simulink model "Prob_8_DONE"  (R2025a)
settings: Solver=ode1  StartTime=0.0  StopTime=12  FixedStep=1/360  RelTol=1e-3
settings Model: Creator=claudelieber  LastModifiedBy=yugpn
settings SolverCC: AlgebraicLoopSolver=TrustRegion
settings DataIOCC: ReturnWorkspaceOutputs=off
settings OptimizationCC: ReuseModelBlockBuffer=off
settings DebuggingCC: UnconnectedInputMsg=warning  UnconnectedOutputMsg=warning  UnconnectedLineMsg=warning  ArithmeticOperatorsInVariantConditions=warning
settings ModelReferenceCC: EnableRefExpFcnMdlSchedulingChecks=on
settings SFSimCC: CustomCodeUndefinedFunction=UseInterfaceOnly
settings RTWCC: GPUComputeCapability=3.5  DLArmComputeVersion=19.05

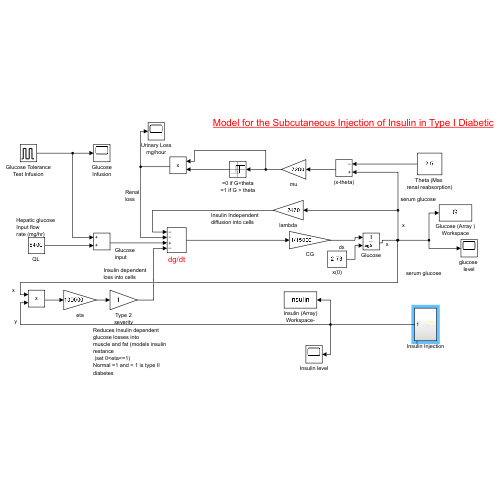
[thumbnail: Simulink's stored preview of the top-level diagram]
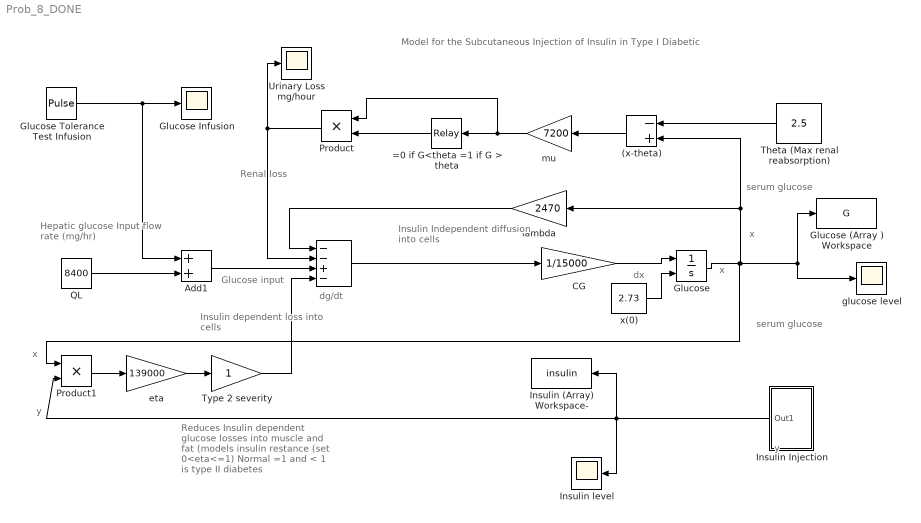
== system Prob_8_DONE ==
  note: Model for the Subcutaneous Injection of Insulin in Type I Diabetic
  note: x
  note: y
  note: y
  note: serum glucose
  note: Reduces Insulin dependent
      | glucose losses into
      | muscle and fat (models insulin
      | restance
      |  (set 0<eta<=1)
      | Normal =1 and < 1 is type II
      | diabetes
  note: x
  note: dx
  note: Insulin dependent
      | loss into cells
  note: serum glucose
  note: dg/dt
  note: Glucose
      | input
  note: x
  note: Renal
      | loss
  note: Insulin Independent
      | diffusion into cells
  note: Hepatic glucose
      | Input flow
      | rate (mg/hr)
  " " : Sum  Inputs=--+-
  (x-theta) : Sum  Inputs=-+
  =0 if G<theta =1 if G > theta : Relay  OnSwitchValue=0  OffSwitchValue=-0.00001
  Add1 : Sum
  CG : Gain  Gain=1/15000
  Glucose : Integrator  InitialConditionSource=external  InitialCondition=0.81
  Glucose Infusion : Scope
      settings: ActiveDisplayYMinimum=-1  ActiveDisplayYMaximum=1  DataLoggingSaveFormat=Array
  Glucose (Array ) Workspace : ToWorkspace  VariableName=G  SampleTime=-1
  Glucose Tolerance Test Infusion : DiscretePulseGenerator  PulseType=Time based  Amplitude=0  Period=10  PulseWidth=5  PhaseDelay=1
  Insulin (Array) Workspace- : ToWorkspace  VariableName=insulin  SampleTime=-1
  Insulin Injection : Subsystem
  Insulin level : Scope
      settings: ActiveDisplayYMinimum=-4.5264238355847652  ActiveDisplayYMaximum=0.89231310643375261  DataLoggingVariableName=ScopeData2  DataLoggingSaveFormat=Array
  Product : Product
  Product1 : Product
  "QL " : Constant  Value=8400
  Theta (Max renal reabsorption) : Constant  Value=2.5
  Type 2 severity : Gain
  Urinary Loss mg/hour : Scope
      settings: ActiveDisplayYMinimum=-1140.6549745940436  ActiveDisplayYMaximum=6361.1676644120716  DataLoggingVariableName=ScopeData3
  "eta " : Gain  Gain=139000
  glucose level : Scope
      settings: ActiveDisplayYMinimum=-26.029411804853417  ActiveDisplayYMaximum=30.5837061812655  DataLoggingSaveFormat=Array
  lambda : Gain  Gain=2470
  mu : Gain  Gain=7200
  x(0) : Constant  Value=2.73
  wires:
  mu/1 -> Product/1, =0 if G<theta =1 if G > theta/1
  " "/1 -> CG/1
  lambda/1 -> " "/1
  Product/1 -> " "/2, Urinary Loss mg/hour/1
  Theta (Max renal reabsorption)/1 -> (x-theta)/1
  x(0)/1 -> Glucose/2
  Glucose/1 -> Product1/1, Glucose (Array ) Workspace/1, glucose level/1, (x-theta)/2, lambda/1
  Product1/1 -> "eta "/1
  Add1/1 -> " "/3
  (x-theta)/1 -> mu/1
  "eta "/1 -> Type 2 severity/1
  =0 if G<theta =1 if G > theta/1 -> Product/2
  Type 2 severity/1 -> " "/4
  CG/1 -> Glucose/1
  "QL "/1 -> Add1/2
  Glucose Tolerance Test Infusion/1 -> Add1/1, Glucose Infusion/1
  Insulin Injection/1(Out1) -> Product1/2, Insulin (Array) Workspace-/1, Insulin level/1

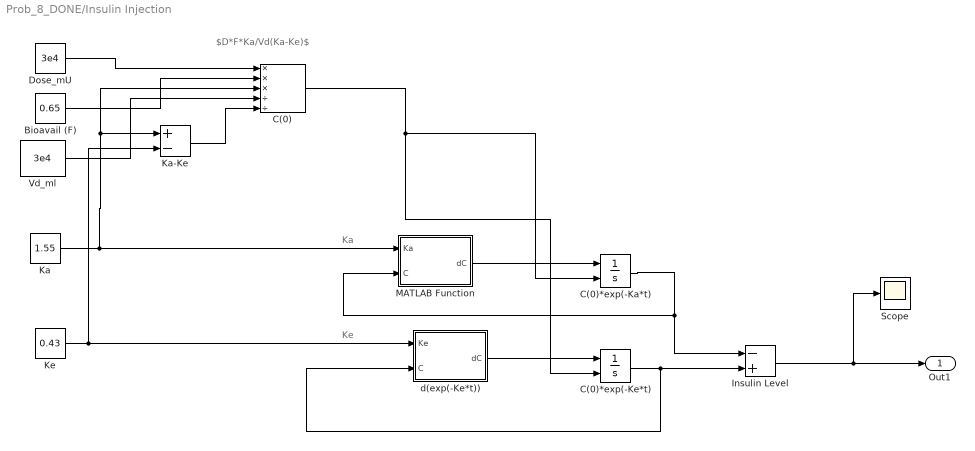
== system Prob_8_DONE/Insulin Injection ==
  note: $D*F*Ka/Vd(Ka-Ke)$
  note: Ke
  note: Ka
  " d(exp(-Ke*t))" : MATLAB Function  TreatAsAtomicUnit=on
  Bioavail (F) : Constant  Value=0.65
  C(0) : Product  Inputs=***//
  C(0)*exp(-Ka*t) : Integrator  InitialConditionSource=external  InitialCondition=1
  C(0)*exp(-Ke*t) : Integrator  InitialConditionSource=external  InitialCondition=1
  Dose_mU : Constant  Value=3e4
  Insulin Level : Sum  Inputs=-+
  Ka : Constant  Value=1.55
  Ka-Ke : Sum  Inputs=+-
  Ke : Constant  Value=0.43
  MATLAB Function : MATLAB Function  TreatAsAtomicUnit=on
  Scope : Scope
      settings: ActiveDisplayYMinimum=-0.049715103610871877  ActiveDisplayYMaximum=0.447435932497847  DataLoggingVariableName=ScopeData4
  Vd_ml : Constant  Value=3e4
  Out1 : Outport  VectorParamsAs1DForOutWhenUnconnected=off
  wires:
  Insulin Level/1 -> Scope/1, Out1/1
  Vd_ml/1 -> C(0)/4
  C(0)/1 -> C(0)*exp(-Ke*t)/2, C(0)*exp(-Ka*t)/2
  " d(exp(-Ke*t))"/1(dC) -> C(0)*exp(-Ke*t)/1
  Ke/1 -> Ka-Ke/2, " d(exp(-Ke*t))"/1(Ke)
  C(0)*exp(-Ke*t)/1 -> " d(exp(-Ke*t))"/2(C), Insulin Level/2
  C(0)*exp(-Ka*t)/1 -> MATLAB Function/2(C), Insulin Level/1
  Ka/1 -> C(0)/3, Ka-Ke/1, MATLAB Function/1(Ka)
  MATLAB Function/1(dC) -> C(0)*exp(-Ka*t)/1
  Dose_mU/1 -> C(0)/1
  Bioavail (F)/1 -> C(0)/2
  Ka-Ke/1 -> C(0)/5

== matlab function Prob_8_DONE/Insulin Injection/ d(exp(-Ke*t)) ==
  data: Ke input; dC output; C input
function dC = fcn(Ke,C)

dC = -Ke*C;

== matlab function Prob_8_DONE/Insulin Injection/MATLAB Function ==
  data: Ka input; dC output; C input
function dC = fcn(Ka,C)

dC = -Ka*C;
